simulink model "L3Pilot_ADF_v1"  (R2018b)
settings: Solver=FixedStepAuto  StartTime=0.0  StopTime=350  RelTol=1e-3  EnableMultiTasking=on
values from neighbouring files (symbols this model uses):
  a_x_MRM_critical = 5    [Var_L3Pilot_ADF_v1.m]
  a_x_MRM_normal = 2    [Var_L3Pilot_ADF_v1.m]
  Distance_forced_lane_change = 10    [Var_L3Pilot_ADF_v1.m]
  K_d_value_100 = 0.09    [Var_L3Pilot_ADF_v1.m]
  K_d_value_130 = 0.08    [Var_L3Pilot_ADF_v1.m]
  K_d_value_60 = 0.1    [Var_L3Pilot_ADF_v1.m]
  K_i_value_100 = 1    [Var_L3Pilot_ADF_v1.m]
  K_i_value_130 = 1    [Var_L3Pilot_ADF_v1.m]
  K_i_value_60 = 1    [Var_L3Pilot_ADF_v1.m]
  K_p_value_100 = 0.1    [Var_L3Pilot_ADF_v1.m]
  K_p_value_130 = 0.1    [Var_L3Pilot_ADF_v1.m]
  K_p_value_60 = 0.1    [Var_L3Pilot_ADF_v1.m]
  K_v1_value_100 = 0.1    [Var_L3Pilot_ADF_v1.m]
  K_v1_value_130 = 0.1    [Var_L3Pilot_ADF_v1.m]
  K_v1_value_60 = 0.1    [Var_L3Pilot_ADF_v1.m]
  K_v2_value_100 = 0.2    [Var_L3Pilot_ADF_v1.m]
  K_v2_value_130 = 0.2    [Var_L3Pilot_ADF_v1.m]
  K_v2_value_60 = 0.2    [Var_L3Pilot_ADF_v1.m]
  Set_velocity = 60/3.6    (= 16.6666666667)    [Var_L3Pilot_ADF_v1.m]
  t_MRM = 60    [Var_L3Pilot_ADF_v1.m]
  t_takeover = 70    [Var_L3Pilot_ADF_v1.m]
  Tabt = 0.1    [Var_L3Pilot_ADF_v1.m]
  x_LC_Forced_value = 99999    [Var_L3Pilot_ADF_v1.m]
undefined symbols (not defined in the file or in its folder): ComponentState
libraries: simulink x2
(part 2 of 2)

== matlab function L3Pilot_ADF_v1/L3Pilot_Mature_ADF_Long/L3Pilot_Mature_ADF_Longitudinal ==
  data: t_abt input; v_t input; v_t_pre input; a_x_t_1 input; a_x_t_1_pre input; a_x_t output; ACC_a_x_req output; I_old output; Set_velocity input; Sensor_DHW_x input; Sensor_DHW_x_pre input; Sensor_delta_v_x input; Sensor_delta_v_x_pre input; a_x_SPL input; ACC_a_x_req_1 input; I_old_1 input; AEB_active_1 input; AEB_counter_1 input; AEB_warning_active_1 input; v_front_veh_pre1 input; a_x_front_pre1 input; K_d input; K_v1 input; K_v2 input; K_p input; K_i input; AEB_active output; AEB_counter output; AEB_warning_active output; v_front_veh_pre output; a_x_front_pre output
function [a_x_t,ACC_a_x_req,I_old,AEB_active,AEB_counter,AEB_warning_active,v_front_veh_pre,a_x_front_pre]  =L3Pilot_Mature_ADF_Long_V1...
    (t_abt,v_t,v_t_pre,a_x_t_1,a_x_t_1_pre,Set_velocity,Sensor_DHW_x,Sensor_DHW_x_pre,...
    Sensor_delta_v_x,Sensor_delta_v_x_pre,a_x_SPL,ACC_a_x_req_1,I_old_1,AEB_active_1,AEB_counter_1,AEB_warning_active_1,v_front_veh_pre1,a_x_front_pre1,...
    K_d,K_v1,K_v2,K_p,K_i)

%%%%%%%%%%%%%%%%%%%%%%%%%%%%%%%%%%%%%%%%%%%%%%%%%%%%%%%%%%%%%%%%%%%%%%%%%%%
v_current = v_t;
a_current = a_x_t_1;
v_requested = Set_velocity;

Obj_x = Sensor_DHW_x-2;

dv_current = Sensor_delta_v_x;

v_front_veh = v_current-dv_current;

T  =t_abt;
I_old_value = I_old_1;

% Consider the acceleration of the front vehicle incl. PT1-Filter to avoid
% to heavy jumps if the predecessor comes to to a standstill. 
if ~isnan(v_front_veh_pre1)
    a_x_front = (v_front_veh-v_front_veh_pre1)./t_abt;
else
    a_x_front = 0;
end
if abs(a_x_front)>15
    a_x_front = 0;
end
if a_x_front>0
    a_x_front = 0;
end

K_PT1_ax = 1;
T_ax = 0.2;
a_x_front_PT1 = T_ax*(K_PT1_ax*a_x_front-a_x_front_pre1)+a_x_front_pre1;

%%%%%%%%%%%%%%%%%%%%%%%%%%%%%%%%%%%%%%%%%%%%%%%%%%%%%%%%%%%%%%%%%%%%%%%%%%%
% ACC Parameters

dx_min= 5 ;%m
timegap = 1.6; %s
THW_react = 8; %s
a_x_max_0 = 3.5; %m/s²
a_x_max_80 = 3 ; %m/s²
a_x_min = -3; %m/s²

a_x_max = interp1([0,80/3.6,999/.36],[a_x_max_0,a_x_max_80,a_x_max_80],v_current);


%%%%%%%%%%%%%%%%%%%%%%%%%%%%%%%%%%%%%%%%%%%%%%%%%%%%%%%%%%%%%%%%%%%%%%%%%%%
% ACC Controll

dv_des = K_d*(timegap * v_current - Obj_x + dx_min);

% Factor applied to the acceleration depends on the time gap to the
% predecessor (the closer the object, the stronger the acceleraiton is
% considered)
current_THW = (Obj_x - dx_min)./v_current;
K_a = min([1,max([0.2,0.2-0.7/(2.5-0.9)*(current_THW-2.5)])]);

if a_x_front_PT1<-1.5
    a_x_front_PT1_in = a_x_front_PT1;
else
    a_x_front_PT1_in = 0;
end

if abs(dv_current)>1
    dv_current_value = dv_current;
else
    dv_current_value = 0;
end

a_des_d = K_v1 * (-1*dv_current_value - dv_des)+ K_a*a_x_front_PT1_in;
% if abs(a_des_d)<0.5
%     a_des_d = 0;
% end

a_des_v = K_v2 * (v_requested - v_current);
% if abs(a_des_v)<0.2
%     a_des_v = 0;
% end

a_des = nanmin([a_des_d, a_des_v]);

if a_des < a_x_max
    a_des_f = a_des;
else
    a_des_f =a_x_max;
end

if a_des_f < a_x_min
    a_des_f =a_x_min;
end

I_new =(a_des_f - a_current) *(K_i * T) + I_old_value;
a_des_PI1 = a_des_f + (a_des_f - a_current)*K_p +I_new ;

a_des_PI = a_des_PI1;

% additional PT1
% a_des_PI_PT1= 0.5*(2*a_des_PI- a_current)+a_current;

% Output
ACC_a_x_req=a_des_PI;
I_old = I_new;

%%%%%%%%%%%%%%%%%%%%%%%%%%%%%%%%%%%%%%%%%%%%%%%%%%%%%%%%%%%%%%%%%%%%%%%%%%%
% AEB Parameters

t_brake_stage_1 = 0.4;
a_x_build_up_velocity_1 = 35;
a_x_build_up_velocity_2 = 35;

if dv_current>0 && Obj_x<200 
    TTC_front = Obj_x./dv_current;
else
    TTC_front =999;
end

x_remain = 0.5;
if dv_current >-0.5
    a_required = min([a_x_t_1_pre,-(dv_current.^2) / (2 * (Obj_x-x_remain))]);
else
    a_required = -1;
end

v_AEB = [0,10,20,30,40,50,60,70,80,90,100,110,120,130,140,150,250]/3.6;
threshold_AEB_warning = [1.2 1.2 1.3 1.4 1.5 1.6 1.7 1.8 1.9 1.9 1.9 1.9 1.9 1.9 1.9 1.9 1.9];

if v_front_veh>1
    % Front vehicle Moving
    threshold_AEB = [0.85 0.85 0.9 0.95 1.1 1.2 1.3 1.4 1.5 1.5 1.5 1.5 1.5 1.5 1.5 1.5 1.5 ];
else
    % Front vehicle stand still
    threshold_AEB = [0.75 0.75 0.8 0.95 1.1 1.2 1.4 1.4 1.4 1.4 1.4 1.4 1.4 1.4 1.4 1.4 1.4];
end

current_threshold_warning = interp1(v_AEB,threshold_AEB_warning,v_current);
current_threshold = interp1(v_AEB,threshold_AEB,v_current);


%%%%%%%%%%%%%%%%%%%%%%%%%%%%%%%%%%%%%%%%%%%%%%%%%%%%%%%%%%%%%%%%%%%%%%%%%%%
% AEB Warning
if TTC_front<current_threshold_warning
    AEB_warning_active = 1;
else
    if a_required>=0 && AEB_warning_active_1==1
        AEB_warning_active = 1;
    else
        AEB_warning_active = 0;
    end
end

%%%%%%%%%%%%%%%%%%%%%%%%%%%%%%%%%%%%%%%%%%%%%%%%%%%%%%%%%%%%%%%%%%%%%%%%%%%
% AEB Control

if TTC_front<current_threshold
   AEB_active = 1;
   AEB_counter = AEB_counter_1+t_abt;
else
   if AEB_active_1 ==1 && a_required>1
        AEB_active = 1;
        AEB_counter = AEB_counter_1+t_abt;
   else
        AEB_active =0;
        AEB_counter = 0;
   end
end

if AEB_active_1 ==1
    if AEB_counter<= t_brake_stage_1
        a_AEB_brake = max([a_x_t_1_pre-a_x_build_up_velocity_1*t_abt,-3.5]);        
    else
        a_AEB_brake = max([a_x_t_1_pre-a_x_build_up_velocity_2*t_abt,a_required,-9.81]);
    end   
else
    a_AEB_brake = NaN;
end

%%%%%%%%%%%%%%%%%%%%%%%%%%%%%%%%%%%%%%%%%%%%%%%%%%%%%%%%%%%%%%%%%%%%%%%%%%%
% Longitudinal Control

% TEST AEB Functionality
% if a_des_PI<0
%     a_des_PI=0;
% end
if AEB_active_1==1
    a_des_PI = 0;
    a_x_SPL = 0;
end

[a_x_t,z_min] = nanmin([a_des_PI,a_x_SPL,a_AEB_brake]);

if z_min==3
    I_old =0;
end

v_front_veh_pre = v_front_veh;
a_x_front_pre = a_x_front_PT1;

== matlab function L3Pilot_ADF_v1/Sensor_Side_lanes/MATLAB Function ==
  data: s_0 input; Distance_front_left output; Distance_rear_left output; Distance_front_right output; Distance_rear_right output; dv_front_left output; dv_rear_left output; dv_front_right output; dv_rear_right output; lane_0 input; v_0 input; s_1 input; lane_1 input; v_1 input; s_2 input; lane_2 input; v_2 input; s_3 input; lane_3 input; v_3 input; s_4 input; lane_4 input; v_4 input; s_5 input; lane_5 input; v_5 input; s_6 input; lane_6 input; v_6 input; s_7 input; lane_7 input; v_7 input; s_8 input; lane_8 input; v_8 input; s_9 input; lane_9 input; v_9 input; s_ego input; lane_ego input; v_ego input; t input
function [Distance_front_left,Distance_rear_left,Distance_front_right,Distance_rear_right,... 
    dv_front_left,dv_rear_left,dv_front_right,dv_rear_right]...
     = Sensor_fusion(s_0,lane_0,v_0,s_1,lane_1,v_1,s_2,lane_2,v_2,s_3,lane_3,v_3,s_4,lane_4,v_4,s_5,lane_5,v_5,...
     s_6,lane_6,v_6,s_7,lane_7,v_7,s_8,lane_8,v_8,s_9,lane_9,v_9,s_ego,lane_ego,v_ego,t)

Distance_front_left = 250;
Distance_rear_left = 250;
Distance_front_right = 250;
Distance_rear_right = 250;

dv_front_left = 0;
dv_rear_left = 0;
dv_front_right = 0; 
dv_rear_right = 0;

rear_offset = 5;

if t>0.1

    Lane_vec_obj = [lane_0,lane_1,lane_2,lane_3,lane_4,lane_5,lane_6,lane_7,lane_8,lane_9];
    s_vec_obj = [s_0,s_1,s_2,s_3,s_4,s_5,s_6,s_7,s_8,s_9];
    v_vec_obj = [v_0,v_1,v_2,v_3,v_4,v_5,v_6,v_7,v_8,v_9];


    delta_lane_vec = Lane_vec_obj-lane_ego;
    delta_s_vec = s_vec_obj;
    delta_v_vec = v_ego-v_vec_obj;

    z_find_obj_left = delta_lane_vec==1;
    z_find_obj_right = delta_lane_vec==-1;

    if sum(z_find_obj_left)>0
        delta_s_left_vec = delta_s_vec(z_find_obj_left);
        delta_v_left_vec = delta_v_vec(z_find_obj_left);

        z_find_pos_left = find(delta_s_left_vec>=0);
        if ~isempty(z_find_pos_left)
            delta_s_left_pos_vec = delta_s_left_vec(z_find_pos_left);
            delta_v_left_pos_vec = delta_v_left_vec(z_find_pos_left);
            [min_delta_s_left_pos_vec,z_min_pos_left] = min(delta_s_left_pos_vec);

            Distance_front_left = min_delta_s_left_pos_vec;
            dv_front_left = delta_v_left_pos_vec(z_min_pos_left);
        end

        z_find_neg_left = find(delta_s_left_vec<0);
        if ~isempty(z_find_neg_left)
            delta_s_left_neg_vec = -1*delta_s_left_vec(z_find_neg_left);
            delta_v_left_neg_vec = delta_v_left_vec(z_find_neg_left);
            [min_delta_s_left_neg_vec,z_min_neg_left] = min(delta_s_left_neg_vec);

            Distance_rear_left = min_delta_s_left_neg_vec-rear_offset;
            dv_rear_left = delta_v_left_neg_vec(z_min_neg_left);
        end  
    end

    if sum(z_find_obj_right)>0
        delta_s_right_vec = delta_s_vec(z_find_obj_right);
        delta_v_right_vec = delta_v_vec(z_find_obj_right);

        z_find_pos_right = find(delta_s_right_vec>=0);
        if ~isempty(z_find_pos_right)
            delta_s_right_pos_vec = delta_s_right_vec(z_find_pos_right);
            delta_v_right_pos_vec = delta_v_right_vec(z_find_pos_right);
            [min_delta_s_right_pos_vec,z_min_pos_right] = min(delta_s_right_pos_vec);

            Distance_front_right = min_delta_s_right_pos_vec;
            dv_front_right = delta_v_right_pos_vec(z_min_pos_right);
        end

        z_find_neg_right = find(delta_s_right_vec<0);
        if ~isempty(z_find_neg_right)
            delta_s_right_neg_vec = -1*delta_s_right_vec(z_find_neg_right);
            delta_v_right_neg_vec = delta_v_right_vec(z_find_neg_right);
            [min_delta_s_right_neg_vec,z_min_neg_right] = min(delta_s_right_neg_vec);

            Distance_rear_right = min_delta_s_right_neg_vec-rear_offset;
            dv_rear_right = delta_v_right_neg_vec(z_min_neg_right);
        end  
    end

end

% Distance_front_left = 250;
% Distance_rear_left = 250;
% Distance_front_right = 250;
% Distance_rear_right = 250;
% 
% dv_front_left = 0;
% dv_rear_left = 0;
% dv_front_right = 0; 
% dv_rear_right = 0;

== matlab function L3Pilot_ADF_v1/Forced_LC_fct ==
  data: t_sim input; x_LC_Forced_value input; Forced_lane_change_status output; Distance_to_lane_end output; x_ego input; LC_Status input; LaneCountLeft input; Distance_forced_lane_change input; Forced_lane_change_status1 input; max_force_lane_change1 input; max_force_lane_change output
function [Forced_lane_change_status,Distance_to_lane_end,max_force_lane_change] = Forced_LC_fct(t_sim,x_LC_Forced_value,x_ego,LC_Status,...
    LaneCountLeft,Distance_forced_lane_change,...
    Forced_lane_change_status1,max_force_lane_change1)

Forced_lane_change_status = 0;

% Distance to lane end --> required for deceleration
if (LaneCountLeft<=1) && (x_ego>= x_LC_Forced_value) && (x_ego<= (x_LC_Forced_value+Distance_forced_lane_change))
   
    Distance_to_lane_end = (x_LC_Forced_value+Distance_forced_lane_change)-x_ego;
    
else
    Distance_to_lane_end =999;
end


% Set max status to zeros; max status is required to check whether a the
% end of lane trigger has been set earlier in the simulation
if t_sim<=5
   max_force_lane_change = 0;
end

% Decide depending on the force lane change status whether the force lane
% change shall be activitated.
if Forced_lane_change_status1==1
    Forced_lane_change_status = Forced_lane_change_status1;
    if abs(LC_Status) >0
        Forced_lane_change_status = 0;
    end
else
    if x_ego> x_LC_Forced_value && x_ego<= (x_LC_Forced_value+Distance_forced_lane_change) ...
            && max_force_lane_change1==0 && LaneCountLeft==0
        Forced_lane_change_status = 1;
    else
        Forced_lane_change_status = 0;
    end
end

% Set new max status in case the current status is higher than the previous
% one
if Forced_lane_change_status>max_force_lane_change1
    max_force_lane_change = Forced_lane_change_status;
else
    max_force_lane_change = max_force_lane_change1;
end
